simulink model "linear_pendulum_model"  (R2024a)
settings: Solver=ode45  StartTime=0.0  StopTime=10  RelTol=1e-3
settings Model: Creator=jeff  LastModifiedBy=jeff

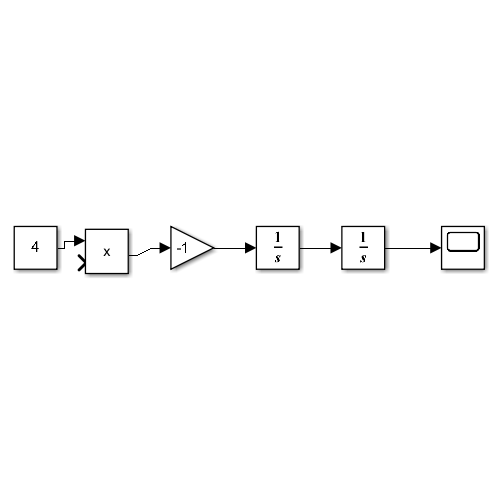
[thumbnail: Simulink's stored preview of the top-level diagram]
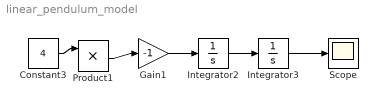
== system linear_pendulum_model ==
  Constant3 : Constant  Value=4
  Gain1 : Gain  Gain=-1
  Integrator2 : Integrator
  Integrator3 : Integrator  InitialCondition=1
  Product1 : Product
  Scope : Scope
  wires:
  Constant3/1 -> Product1/1
  Product1/1 -> Gain1/1
  Gain1/1 -> Integrator2/1
  Integrator2/1 -> Integrator3/1
  Integrator3/1 -> Scope/1
